simulink model "q_maglev_piv"  (Simulink 7.7)
settings: Solver=ode4  StartTime=0.0  StopTime=inf  FixedStep=0.002  RelTol=1e-3  AbsTol=1e-6
values from neighbouring files (symbols this model uses):
  IC_MAX = 3    [config_maglev.m]
  K_AMP = 3    [setup_maglev.m]
  K_B = Tb / 5    (= 0.0028)    [config_maglev.m]
  Kff_b = ic0 / xb0    [d_maglev_pi_piv.m]    (also in setup_maglev.m = 0)
  Ki_b = -p0*wn_b^2*ic0/(2*g)    [d_maglev_pi_piv.m]    (also in setup_maglev.m = 0)
  Ki_c = wn_c^2 * tau_c / Kc_dc    [d_maglev_pi_piv.m]    (also in setup_maglev.m = 0)
  Kp_b = -(2*p0*zeta_b*wn_b*xb0 + wn_b^2*xb0+2*g)*ic0/(2*xb0*g)    [d_maglev_pi_piv.m]    (also in setup_maglev.m = 0)
  Kp_c = (2*zeta_c*wn_c*tau_c - 1) / Kc_dc    [d_maglev_pi_piv.m]    (also in setup_maglev.m = 0)
  Kv_b = -(p0+2*zeta_b*wn_b)*ic0/(2*g)    [d_maglev_pi_piv.m]    (also in setup_maglev.m = 0)
  MAX_XB_WDUP = 1    [setup_maglev.m]
  Rs = 1    [config_maglev.m]
  Tb = 0.014    [config_maglev.m]
  VMAX_AMP = 24    [config_maglev.m]
  wcf = 2 * pi * 75    (= 471.238898038)    [setup_maglev.m]
  xb0 = 6e-3    (= 0.006)    [setup_maglev.m]
  XB_REF_RATE = 5e-3    (= 0.005)    [setup_maglev.m]
  zetaf = 0.9    [setup_maglev.m]
undefined symbols (not defined in the file or in its folder): HIL, qc_get_step_size
libraries: quarc_library x3, simulink x1
settings Model: Creator=MLevis  LastModifiedBy=MLevis  SimulationMode=external  ExtModeTrigDuration=10000  ExtModeAutoUpdateStatusClock=off  BufferReuse=off
settings SolverCC: PositivePriorityOrder=on
settings DataIOCC: LimitDataPoints=off
settings OptimizationCC: BooleanDataType=off  OptimizeBlockIOStorage=off  BufferReuse=off  ExpressionFolding=off  FoldNonRolledExpr=off  LocalBlockOutputs=off  InitFltsAndDblsToZero=on
settings DebuggingCC: SaveWithParameterizedLinksMsg=none  SignalResolutionControl=TryResolveAllWithWarning  SolverPrmCheckMsg=none  MultiTaskDSMMsg=warning  MultiTaskCondExecSysMsg=none  StrictBusMsg=None
settings HardwareCC: TargetHWDeviceType=32-bit Generic
settings RTWCC: SystemTargetFile=quarc_win64.tlc  TemplateMakefile=quarc_default_tmf  Description=QUARC Win64 Target  ProcessScript=quarc_win64_make_rtw_hook  IncludeERTFirstTime=on
settings STFCustomTargetCC: TargetPreCompLibLocation=C:\PROGRA~3\QUARC\lib\2011a\win64\release  FunctionExecutionProfile=off  GeneratePreprocessorConditionals=Disable all  SystemTargetFile=quarc_win64.tlc
settings GRTTargetCC: TargetPreCompLibLocation=C:\PROGRA~3\QUARC\lib\2011a\win64\release  ParMdlRefBuildCompliant=off  CompOptLevelCompliant=off  MatFileLogging=off  ExtMode=on  ExtModeMexFile=quarc_comm

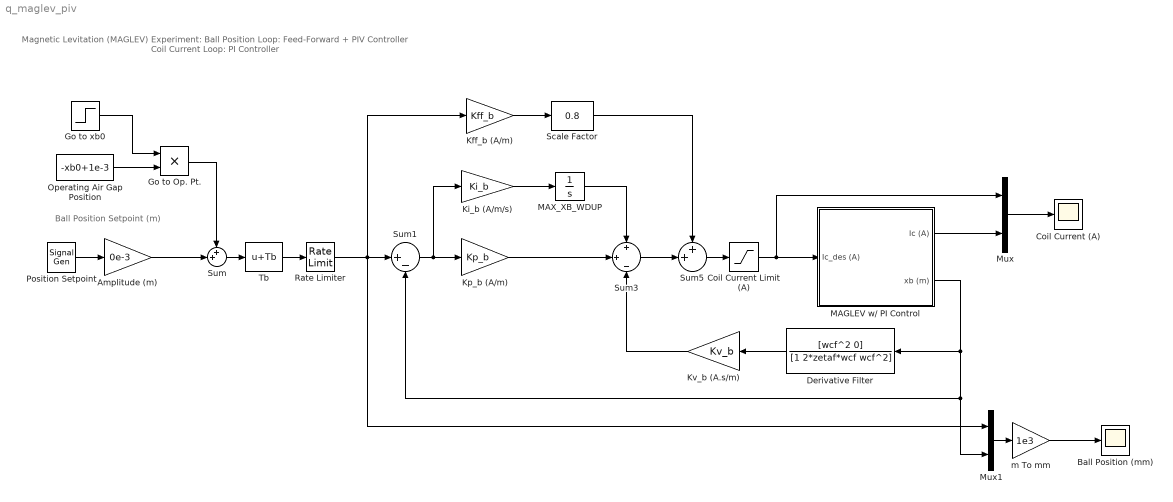
== system q_maglev_piv ==
  note: Magnetic Levitation (MAGLEV) Experiment:
      | Ball Position Loop: Feed-Forward + PIV Controller
      | Coil Current Loop: PI Controller
  note: Ball Position Setpoint (m)
  Amplitude (m) : Gain  Gain=0e-3  SaturateOnIntegerOverflow=on  OutDataTypeStr=Inherit: Same as input  ParamDataTypeStr=Inherit: Same as input
  Ball Position (mm) : Scope
      settings: TimeRange=10  YMin=0  YMax=15  SaveName=data_xb  DataFormat=Array
  Coil Current Limit (A) : Saturate  UpperLimit=IC_MAX  LowerLimit=0
  Coil Current (A) : Scope
      settings: TimeRange=10  YMin=-0.25  YMax=3  SaveName=data_Ic  DataFormat=Array
  Derivative Filter : TransferFcn  Numerator=[wcf^2 0]  Denominator=[1 2*zetaf*wcf wcf^2]
  Go to Op. Pt. : Product  RndMeth=Zero
  Go to xb0 : Step  Time=2  SampleTime=0
  Kff_b (A/m) : Gain  Gain=Kff_b  SaturateOnIntegerOverflow=on  OutDataTypeStr=Inherit: Same as input  ParamDataTypeStr=Inherit: Same as input
  Ki_b (A/m/s) : Gain  Gain=Ki_b  SaturateOnIntegerOverflow=on  OutDataTypeStr=Inherit: Same as input  ParamDataTypeStr=Inherit: Same as input
  Kp_b (A/m) : Gain  Gain=Kp_b  SaturateOnIntegerOverflow=on  OutDataTypeStr=Inherit: Same as input  ParamDataTypeStr=Inherit: Same as input
  Kv_b (A.s/m) : Gain  Gain=Kv_b  SaturateOnIntegerOverflow=on  OutDataTypeStr=Inherit: Same as input  ParamDataTypeStr=Inherit: Same as input
  MAGLEV w/ PI Control : Subsystem
  MAX_XB_WDUP : Integrator  LimitOutput=on  UpperSaturationLimit=MAX_XB_WDUP  LowerSaturationLimit=- MAX_XB_WDUP
  Mux : Mux  Inputs=2
  Mux1 : Mux  Inputs=2
  Operating Air Gap Position : Constant  Value=-xb0+1e-3
  Position Setpoint : SignalGenerator  WaveForm=square  Frequency=.25
  Rate Limiter : RateLimiter  RisingSlewLimit=XB_REF_RATE  FallingSlewLimit=-XB_REF_RATE  SampleTimeMode=inherited
  Scale Factor : simulink/Math Operations/Slider Gain  SystemSampleTime=-1  low=0  gain=0.8  high=1
  Sum : Sum  Inputs=++|
  Sum1 : Sum  Inputs=|+-  SaturateOnIntegerOverflow=on  InputSameDT=on  OutDataTypeStr=Inherit: Same as first input
  Sum3 : Sum  Inputs=+|+|-  SaturateOnIntegerOverflow=on  InputSameDT=on  OutDataTypeStr=Inherit: Same as first input
  Sum5 : Sum  Inputs=++|  SaturateOnIntegerOverflow=on  InputSameDT=on  OutDataTypeStr=Inherit: Same as first input
  Tb : Bias  Bias=Tb
  m To mm : Gain  Gain=1e3  SaturateOnIntegerOverflow=on  OutDataTypeStr=Inherit: Same as input  ParamDataTypeStr=Inherit: Same as input
  wires:
  Sum1/1 -> Ki_b (A/m/s)/1, Kp_b (A/m)/1
  Mux1/1 -> m To mm/1
  Ki_b (A/m/s)/1 -> MAX_XB_WDUP/1
  MAX_XB_WDUP/1 -> Sum3/1
  Kp_b (A/m)/1 -> Sum3/2
  Sum3/1 -> Sum5/2
  Kv_b (A.s/m)/1 -> Sum3/3
  Kff_b (A/m)/1 -> Scale Factor/1
  MAGLEV w/ PI Control/1(Ic (A)) -> Mux/2
  Coil Current Limit (A)/1 -> MAGLEV w/ PI Control/1(Ic_des (A)), Mux/1
  Sum5/1 -> Coil Current Limit (A)/1
  m To mm/1 -> Ball Position (mm)/1
  Mux/1 -> Coil Current (A)/1
  Derivative Filter/1 -> Kv_b (A.s/m)/1
  Rate Limiter/1 -> Sum1/1, Kff_b (A/m)/1, Mux1/1
  Position Setpoint/1 -> Amplitude (m)/1
  Sum/1 -> Tb/1
  MAGLEV w/ PI Control/2(xb (m)) -> Derivative Filter/1, Mux1/2, Sum1/2
  Amplitude (m)/1 -> Sum/2
  Operating Air Gap Position/1 -> Go to Op. Pt./2
  Go to Op. Pt./1 -> Sum/1
  Go to xb0/1 -> Go to Op. Pt./1
  Scale Factor/1 -> Sum5/1
  Tb/1 -> Rate Limiter/1

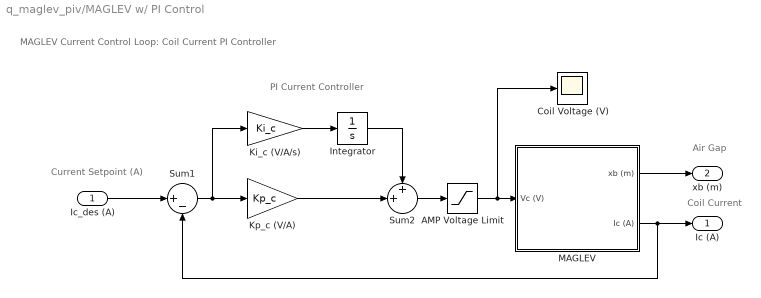
== system q_maglev_piv/MAGLEV w/ PI Control ==
  note: MAGLEV Current Control Loop:
      | Coil Current PI Controller
  note: Current Setpoint (A)
  note: PI Current Controller
  note: Coil Current
  note: Air Gap
  Ic_des (A) : Inport
  AMP Voltage Limit : Saturate  UpperLimit=VMAX_AMP  LowerLimit=-VMAX_AMP
  Coil Voltage (V) : Scope
      settings: TimeRange=10  YMin=-25  YMax=25  SaveName=data_Vc  DataFormat=Array
  Integrator : Integrator  LimitOutput=on  UpperSaturationLimit=VMAX_AMP  LowerSaturationLimit=-VMAX_AMP
  Ki_c (V/A/s) : Gain  Gain=Ki_c  SaturateOnIntegerOverflow=on  OutDataTypeStr=Inherit: Same as input  ParamDataTypeStr=Inherit: Same as input
  Kp_c (V/A) : Gain  Gain=Kp_c  SaturateOnIntegerOverflow=on  OutDataTypeStr=Inherit: Same as input  ParamDataTypeStr=Inherit: Same as input
  MAGLEV : Subsystem
  Sum1 : Sum  Inputs=|+-  SaturateOnIntegerOverflow=on  InputSameDT=on  OutDataTypeStr=Inherit: Same as first input
  Sum2 : Sum  Inputs=++|  SaturateOnIntegerOverflow=on  InputSameDT=on  OutDataTypeStr=Inherit: Same as first input
  Ic (A) : Outport  InitialOutput=0
  xb (m) : Outport  Port=2  InitialOutput=0
  wires:
  Sum1/1 -> Kp_c (V/A)/1, Ki_c (V/A/s)/1
  Kp_c (V/A)/1 -> Sum2/2
  Sum2/1 -> AMP Voltage Limit/1
  Integrator/1 -> Sum2/1
  AMP Voltage Limit/1 -> Coil Voltage (V)/1, MAGLEV/1(Vc (V))
  Ic_des (A)/1 -> Sum1/1
  Ki_c (V/A/s)/1 -> Integrator/1
  MAGLEV/1(xb (m)) -> xb (m)/1
  MAGLEV/2(Ic (A)) -> Sum1/2, Ic (A)/1

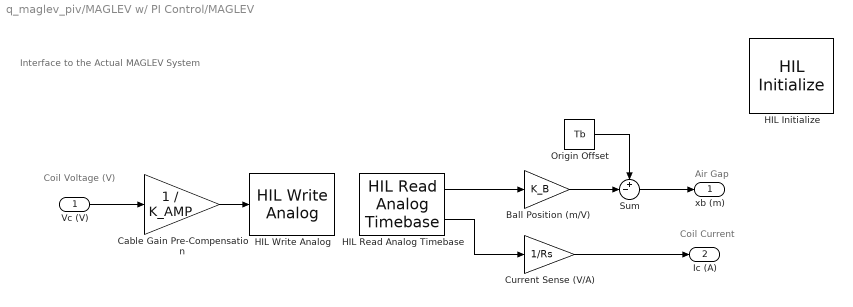
== system q_maglev_piv/MAGLEV w/ PI Control/MAGLEV ==
  note: Interface to the Actual
      | MAGLEV System
  note: Coil Current
  note: Air Gap
  note: Coil Voltage (V)
  Vc (V) : Inport
  Ball Position (m/V) : Gain  Gain=K_B  SaturateOnIntegerOverflow=on  OutDataTypeStr=Inherit: Same as input  ParamDataTypeStr=Inherit: Same as input
  Cable Gain Pre-Compensation : Gain  Gain=1 / K_AMP  SaturateOnIntegerOverflow=on  OutDataTypeStr=Inherit: Same as input  ParamDataTypeStr=Inherit: Same as input
  Current Sense (V/A) : Gain  Gain=1/Rs  SaturateOnIntegerOverflow=on  OutDataTypeStr=Inherit: Same as input  ParamDataTypeStr=Inherit: Same as input
  HIL Initialize : quarc_library/Data Acquisition/Generic/Configuration/HIL Initialize  object_name=HIL-1  board_type=q2_usb  board_number=0  board_options=d0=digital;d1=digital;led=auto;update_rate=normal;decimation=1  exclusive=off  active=off  hardware_clocks=[0:2]  clock_modes=[]  initial_clock_frequencies=[]  set_clock_params_at_start=off  set_clock_params_at_switch_in=off  set_clock_frequencies_at_start=off  set_clock_frequencies_at_switch_in=off  analog_input_channels=[0:1]  analog_input_maximums=10  analog_input_minimums=-10  set_analog_input_params_at_start=on  set_analog_input_params_at_switch_in=off  analog_output_channels=[0:1]  analog_output_maximums=10  analog_output_minimums=-10  initial_analog_outputs=[0]  final_analog_outputs=[0]  watchdog_analog_outputs=0  set_analog_output_params_at_start=on  set_analog_output_params_at_switch_in=off  set_analog_outputs_at_start=on  set_analog_outputs_at_switch_in=off  set_analog_outputs_at_terminate=on  set_analog_outputs_at_switch_out=off  set_analog_outputs_on_watchdog=off  digital_input_channels=[]  digital_output_channels=[]  digital_output_configuration=[]  initial_digital_outputs=[1]  final_digital_outputs=[1]  watchdog_digital_outputs=[1]  set_digital_output_params_at_start=off  set_digital_output_params_at_switch_in=off  set_digital_outputs_at_start=on  set_digital_outputs_at_switch_in=off  set_digital_outputs_at_terminate=on  set_digital_outputs_at_switch_out=off  set_digital_outputs_on_watchdog=off  encoder_channels=[0:1]  quadrature=[4]  encoder_filter_frequency=[]  initial_encoder_counts=[0]  set_encoder_params_at_start=on  set_encoder_params_at_switch_in=off  set_encoder_counts_at_start=on  set_encoder_counts_at_switch_in=off  pwm_channels=[]  pwm_modes=[0]  pwm_frequency=1/0.020  pwm_configuration=[]  pwm_alignment=[]  pwm_polarity=[]  pwm_leading_deadband=[]  pwm_trailing_deadband=[]  initial_pwm_outputs=[0]  final_pwm_outputs=[0]  watchdog_pwm_outputs=[0]  set_pwm_params_at_start=on  set_pwm_params_at_switch_in=off  set_pwm_outputs_at_start=on  set_pwm_outputs_at_switch_in=off  set_pwm_outputs_at_terminate=on  set_pwm_outputs_at_switch_out=off  set_pwm_outputs_on_watchdog=off  other_output_channels=[]  initial_other_outputs=[]  final_other_outputs=[]  watchdog_other_outputs=[]  set_other_outputs_at_start=off  set_other_outputs_at_switch_in=off  set_other_outputs_at_terminate=off  set_other_outputs_at_switch_out=off  set_other_outputs_on_watchdog=off
  HIL Read Analog Timebase : quarc_library/Data Acquisition/Generic/Timebases/HIL Read Analog Timebase  object_name=HIL-1  clock=0  channels=[0:1]  samples_in_buffer=max(ceil(1/qc_get_step_size), 1)  active=on  vector_output=off
      settings: AttributesFormatString=(%<object_name>)
  HIL Write Analog : quarc_library/Data Acquisition/Generic/Immediate I//O/HIL Write Analog  object_name=HIL-1  channels=0  sample_time=-1  active=off  vector_input=off
  Origin Offset : Constant  Value=Tb
  Sum : Sum  Inputs=+-|
  xb (m) : Outport  InitialOutput=0
  Ic (A) : Outport  Port=2  InitialOutput=0
  wires:
  Current Sense (V/A)/1 -> Ic (A)/1
  Cable Gain Pre-Compensation/1 -> HIL Write Analog/1
  HIL Read Analog Timebase/2 -> Current Sense (V/A)/1
  Origin Offset/1 -> Sum/1
  Ball Position (m/V)/1 -> Sum/2
  HIL Read Analog Timebase/1 -> Ball Position (m/V)/1
  Sum/1 -> xb (m)/1
  Vc (V)/1 -> Cable Gain Pre-Compensation/1
